simulink model "DCDC_BBC_hybrid2"  (R2021a)
settings: Solver=VariableStepAuto  StartTime=0.0  StopTime=10.0  RelTol=1e-3
values from neighbouring files (symbols this model uses):
  C_capacitance = 40e-3    (= 0.04)    [Hybrid1.m]    (also in Hybrid2.m; PID.m; PPO.m)
  error_threshold = 0.02    [Hybrid1.m]    (also in Hybrid2.m; PPO.m = 0.1)
  init_action = 1    [Hybrid1.m]    (also in Hybrid2.m; PID.m; PPO.m)
  L_inductance = 10e-6    (= 1e-05)    [Hybrid1.m]    (also in Hybrid2.m; PID.m; PPO.m)
  R_load = 100    [Hybrid1.m]    (also in Hybrid2.m; PID.m; PPO.m)
  stopping_criterion = 1000    [Hybrid1.m]    (also in Hybrid2.m; PPO.m = 500)
  V_ref = 110    [Hybrid1.m]    (also in Hybrid2.m; PID.m = 30; PPO.m = 80)
  V_source_value = 48    [Hybrid1.m]    (also in Hybrid2.m; PID.m; PPO.m)
undefined symbols (not defined in the file or in its folder): rl
libraries: spsSeriesRLCBranchLib x3, spsDiodeLib x1, spsMosfetLib x1, spsDCVoltageSourceLib x1, spsVoltageMeasurementLib x1, spspowerguiLib x1, rllib x1
settings Model: Creator=krupa  LastModifiedBy=krupa

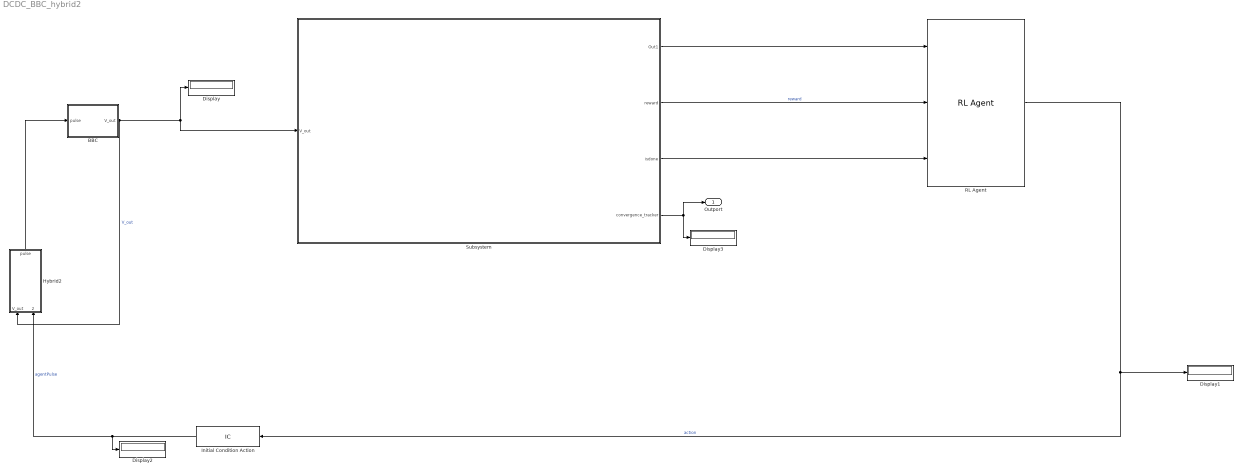
== system DCDC_BBC_hybrid2 ==
  BBC : Subsystem
  Display{,1..3} (4 alike) : Display
  Hybrid2 : Subsystem
  Initial Condition Action : InitialCondition  Value=init_action
  RL Agent : rllib/RL Agent  Agent=rl.util.PolicyInstance.get('DCDC_BBC_RL/RL Agent')  ExternalActionAsInput=off  ProvideCumRwd=off  TreatAsDirectFeedthrough=on
  Subsystem : Subsystem
  Outport : Outport
  wires:
  Subsystem/4(convergence_tracker) -> Display3/1, Outport/1
  RL Agent/1 -> Initial Condition Action/1, Display1/1  "action"
  Subsystem/1(Out1) -> RL Agent/1
  Subsystem/3(isdone) -> RL Agent/3
  BBC/1(V_out) -> Hybrid2/1(V_out), Display/1, Subsystem/1(V_out)  "V_out"
  Initial Condition Action/1 -> Hybrid2/2(agentPulse), Display2/1  "agentPulse"
  Subsystem/2(reward) -> RL Agent/2  "reward"
  Hybrid2/1(pulse) -> BBC/1(pulse)

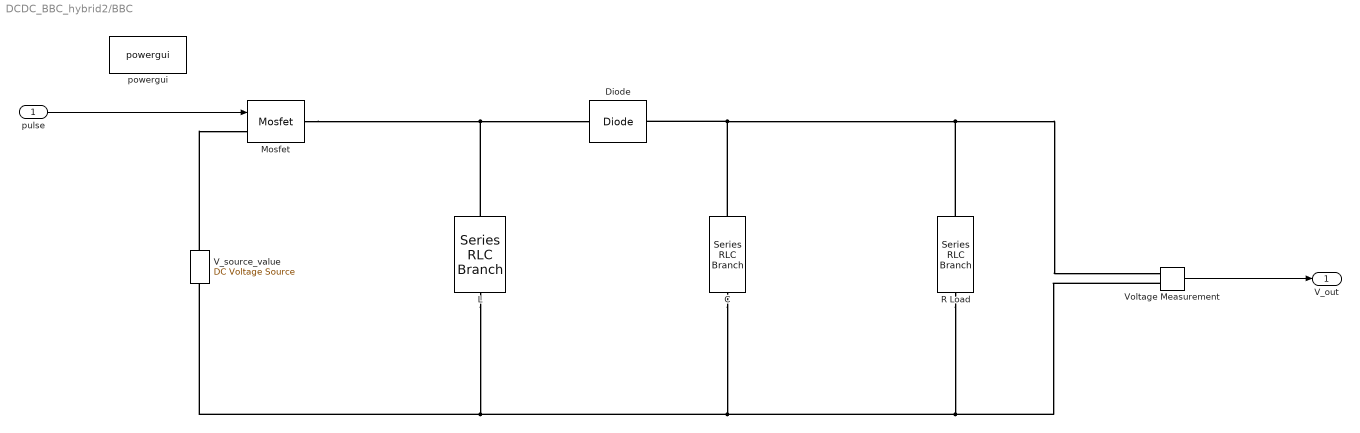
== system DCDC_BBC_hybrid2/BBC ==
  pulse : Inport
  C : spsSeriesRLCBranchLib/Series RLC Branch  LConnTagsString=__new0  RConnTagsString=__new0  BranchType=C  Resistance=1  Inductance=1e-3  SetiL0=off  InitialCurrent=0  Capacitance=C_capacitance  Setx0=off  InitialVoltage=0  Measurements=None
  Diode : spsDiodeLib/Diode  Ron=0.001  Lon=0  Vf=0.8  IC=0  UseSnubber=0  Rs=500  Cs=250e-9  Measurements=off
  L : spsSeriesRLCBranchLib/Series RLC Branch  LConnTagsString=__new0  RConnTagsString=__new0  BranchType=L  Resistance=1  Inductance=L_inductance  SetiL0=off  InitialCurrent=0  Capacitance=1e-6  Setx0=off  InitialVoltage=0  Measurements=None
  Mosfet : spsMosfetLib/Mosfet  Ron=0.1  Lon=0  Rd=0.01  Vfd=0  IC=0  Rs=1e5  Cs=inf  Measurements=off
  R Load : spsSeriesRLCBranchLib/Series RLC Branch  LConnTagsString=__new0  RConnTagsString=__new0  BranchType=R  Resistance=R_load  Inductance=1e-3  SetiL0=off  InitialCurrent=0  Capacitance=1e-6  Setx0=off  InitialVoltage=0  Measurements=None
  V_source_value : spsDCVoltageSourceLib/DC Voltage Source  Amplitude=V_source_value  Measurements=None
  Voltage Measurement : spsVoltageMeasurementLib/Voltage Measurement  PhasorSimulation=off  OutputType=Complex  PSBequivalent=0
  powergui : spspowerguiLib/powergui  Priority=1  SimulationMode=Continuous  SampleTime=50e-6  frequency=60  Iterations=50  frequencyindice=0  Pbase=100e6  ErrMax=1e-4  UnitsV=kV  UnitsW=MW  buscounter=0  FunctionMessages=off  echomessages=off  EnableUseOfTLC=off  CurrentSourceSwitches=off  DisableSnubberDevices=off  DisableRonSwitches=off  DisableVfSwitches=off  DisplayEquations=off  AutomaticDiscreteSolvers=off  SolverType=Tustin/Backward Euler (TBE)  Interpol=off  ExternalGateDelay=off  methode=off  Ts=100  x0status=blocks  SPID=on  SwTol=0  HookPort=off  NonlinearTolerance=1e-4  nMaxIteration=100  ContinueOnMaxIteration=off  RestoreLinks=warning  ResistiveCurrentMeasurement=off  Frange=[0:2:500]  Ylog=off  Xlog=on  ShowGrid=off  save=off  variable=ZData  structure=0  ZoomFFT=off  StartTime=0.0  cycles=1  DisplayStyle=1  fundamental=60  FreqAxis=off  MaxFrequency=1000  frequencyindicesteady=1  RmsSteady=1  display=off
  V_out : Outport
  wires:
  Voltage Measurement/1 -> V_out/1
  pulse/1 -> Mosfet/1
  connections:
  V_source_value/RConn1 -- Mosfet/LConn1
  C/RConn1 -- Voltage Measurement/LConn1 -- R Load/RConn1 -- Diode/LConn1
  L/RConn1 -- Diode/RConn1 -- Mosfet/RConn1
  R Load/LConn1 -- Voltage Measurement/LConn2 -- C/LConn1 -- L/LConn1 -- V_source_value/LConn1

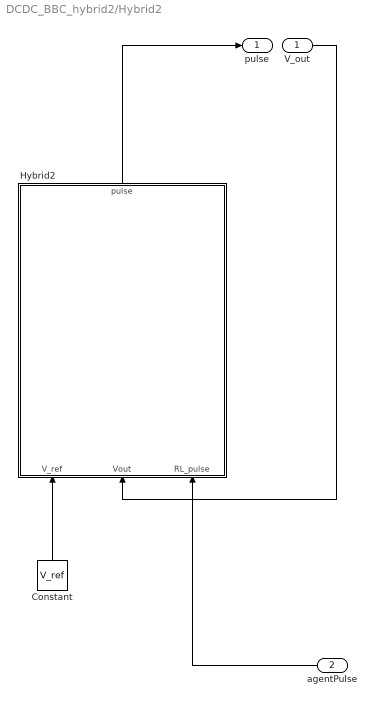
== system DCDC_BBC_hybrid2/Hybrid2 ==
  V_out : Inport
  agentPulse : Inport  Port=2
  Constant : Constant  Value=V_ref
  Hybrid2 : MATLAB Function  TreatAsAtomicUnit=on
  pulse : Outport
  wires:
  Constant/1 -> Hybrid2/1(V_ref)
  Hybrid2/1(pulse) -> pulse/1
  agentPulse/1 -> Hybrid2/3(RL_pulse)
  V_out/1 -> Hybrid2/2(Vout)

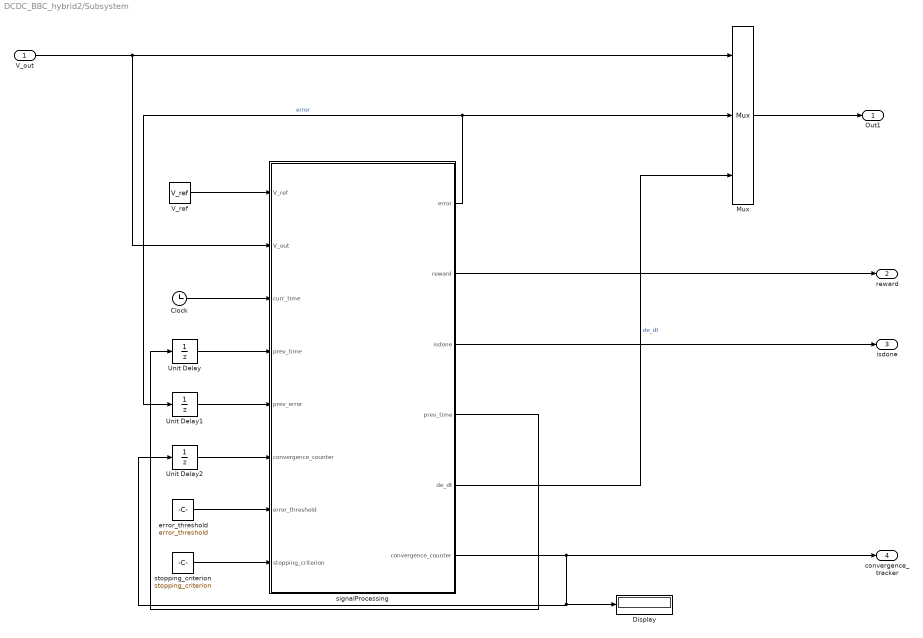
== system DCDC_BBC_hybrid2/Subsystem ==
  V_out : Inport
  Clock : Clock
  Display : Display
  Mux : Mux  Inputs=3
  Unit Delay : UnitDelay  SampleTime=-1  HasFrameUpgradeWarning=on
  Unit Delay1 : UnitDelay  SampleTime=-1  HasFrameUpgradeWarning=on
  Unit Delay2 : UnitDelay  SampleTime=-1  HasFrameUpgradeWarning=on
  V_ref : Constant  Value=V_ref
  error_threshold : Constant  Value=error_threshold
  signalProcessing : MATLAB Function  TreatAsAtomicUnit=on
  stopping_criterion : Constant  Value=stopping_criterion
  Out1 : Outport
  reward : Outport  Port=2
  isdone : Outport  Port=3
  convergence_tracker : Outport  Port=4
  wires:
  signalProcessing/3(isdone) -> isdone/1
  signalProcessing/6(convergence_counter) -> convergence_tracker/1, Unit Delay2/1, Display/1
  signalProcessing/4(prev_time) -> Unit Delay/1
  Unit Delay/1 -> signalProcessing/4("prev_time ")
  Clock/1 -> signalProcessing/3(curr_time)
  signalProcessing/2(reward) -> reward/1
  signalProcessing/1(error) -> Unit Delay1/1, Mux/2  "error"
  Unit Delay2/1 -> signalProcessing/6("convergence_counter ")
  V_out/1 -> Mux/1, signalProcessing/2(V_out)
  V_ref/1 -> signalProcessing/1(V_ref)
  Unit Delay1/1 -> signalProcessing/5(prev_error)
  signalProcessing/5(de_dt) -> Mux/3  "de_dt"
  stopping_criterion/1 -> signalProcessing/8(stopping_criterion)
  error_threshold/1 -> signalProcessing/7(error_threshold)
  Mux/1 -> Out1/1

== matlab function DCDC_BBC_hybrid2/Subsystem/signalProcessing ==
  data: V_ref input; error output; V_out input; curr_time input; prev_time input; prev_error input; convergence_counter input; error_threshold input; stopping_criterion input; reward output; isdone output; prev_time output; de_dt output; convergence_counter output
function [error, reward, isdone, prev_time, de_dt, convergence_counter] = signalProcessing(V_ref, V_out, curr_time, prev_time, prev_error, convergence_counter, error_threshold, stopping_criterion)
%error
abs_Vout = abs(V_out);
error = V_ref - abs_Vout;
abs_error = abs(error);

% change in error
de_dt = (abs_error - abs(prev_error))/(curr_time - prev_time);


if abs_Vout>(V_ref*1.04)
    isdone=1;
else
    isdone = 0;
end

prev_time = curr_time; 

V_ref_lowerBound = V_ref - (V_ref*error_threshold);
V_ref_upperBound = V_ref + (V_ref*error_threshold);
change_error = abs_error - abs(prev_error);


if abs_Vout>=V_ref
    convergence_counter = 1;
end


if ((abs_Vout>V_ref_upperBound)|| (abs_Vout<V_ref_lowerBound && convergence_counter==1))
    reward = -1;
else 
    reward = 1/(abs_error);
end

== matlab function DCDC_BBC_hybrid2/Hybrid2/Hybrid2 ==
  data: V_ref input; pulse output; Vout input; RL_pulse input
function pulse = fcn(V_ref, Vout, RL_pulse)
if abs(Vout)>=V_ref
    pulse = 0;
else
    pulse = RL_pulse;
end
